simulink model "switch_5_24_TN0104"  (R2016b)
settings: Solver=VariableStepAuto  StartTime=0.0  StopTime=0.001  FixedStep=0.001  MaxStep=400e-9  RelTol=1e-3
libraries: fl_lib x9, nesl_utility x4, elec_lib x2
settings Model: Creator=piotr  LastModifiedBy=piotr

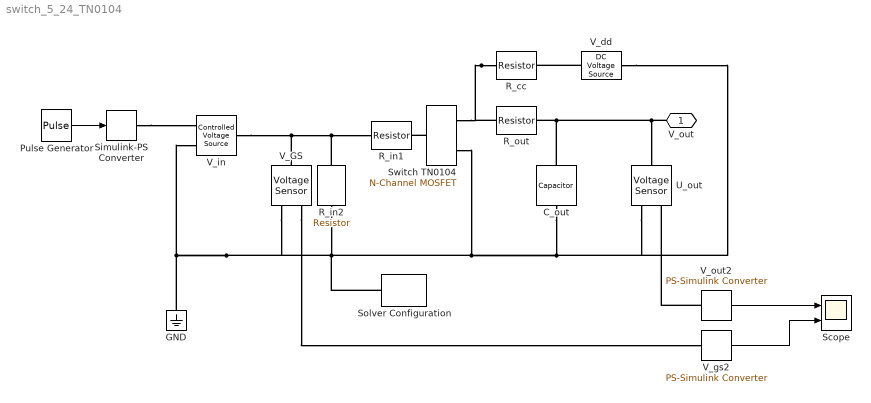
== system switch_5_24_TN0104 ==
  C_out : elec_lib/Passive Devices/Capacitor  enable_table=0  c=10 pF  Cvec=[ 1e-5 1e-6 ] F  Vvec=[ 0 10 ] V  CV_table_symmetry=1  C_tol=5  enable_C_tol=0  tol_distribution=1  nSigma=4  r=1e-6 Ohm  g=0 1/Ohm  initV=0 V  enable_operating_limits=0  operating_limit_action=2  max_working_voltage_range=[ -25 25 ] V  power_rating=1 W  enable_faults=0  fault_action=1  Cscale_faulted=100  R_faulted=0.001 Ohm  G_faulted=0 1/Ohm  tau_fault=0.001 s  enable_temporal_fault=0  t_fault=1 s  enable_behavioral_fault=0  max_permissible_voltage_range=[ -100 100 ] V  t_fail_on_voltage=1 s
  GND : fl_lib/Electrical/Electrical Elements/Electrical Reference
  Pulse Generator : DiscretePulseGenerator  PulseType=Time based  Amplitude=4.5  Period=0.0004  PulseWidth=50
  R_cc : fl_lib/Electrical/Electrical Elements/Resistor  R=2700 Ohm  i_specify=off  i_priority=None  i=0 A  v_specify=off  v_priority=None  v=0 V
  R_in1 : fl_lib/Electrical/Electrical Elements/Resistor  R=1 kOhm  i_specify=off  i_priority=None  i=0 A  v_specify=off  v_priority=None  v=0 V
  R_in2 : fl_lib/Electrical/Electrical Elements/Resistor  R=100 kOhm  i_specify=off  i_priority=None  i=0 A  v_specify=off  v_priority=None  v=0 V
  R_out : fl_lib/Electrical/Electrical Elements/Resistor  R=1 kOhm  i_specify=off  i_priority=None  i=0 A  v_specify=off  v_priority=None  v=0 V
  Scope : Scope  NumInputPorts=2
  Simulink-PS Converter : nesl_utility/Simulink-PS Converter  PhysicalDomain=network_engine_domain  SubClassName=ps_input  LeftPortType=input  RightPortType=output  PseudoPeriodic=off  Frequencies=[]  NoiseDistribution=none  NoiseParameters=[]  Unit=1  AffineConversion=off  InputFiltering=off  SimscapeFilterOrder=1  InputFilterTimeConstant=0.001  UdotUserProvided=1
  Solver Configuration : nesl_utility/Solver Configuration  PhysicalDomain=network_engine_domain  SubClassName=solver  LeftPortType=input  RightPortType=generic  Accelerate=off  Tones=[]  Harmonics=[]  SimulateNoise=off  Profile=off  UseLocalSampling=off  EnableSwitchedLinearOptims=on  FrequencyDomain=off  UseCCode=off  RelTol=0.001  AbsTol=1e-06  MinStep=1e-09  ToWorkspace=off  RevertToSquareIcSolve=off  NumHomotopyIterations=100  PhasorMode=off  PhasorModeNumHarmonics=1  OverrideAbsTol=off  DoDC=off  ResidualTolerance=1e-9  UseLocalSolver=off  LocalSolverChoice=NE_TRAPEZOIDAL_ADVANCER  LocalSolverSampleTime=0.0001  DoFixedCost=off  MaxNonlinIter=3  MaxModeIter=2  LinearAlgebra=Sparse  DelaysMemoryBudget=1024  AutomaticFiltering=on  FilteringTimeConstant=0.001
  Switch TN0104 : elec_lib/Semiconductor Devices/N-Channel MOSFET  parameterization=1  prmDatasheet=1  prmEquCoeff=1  Beta=5 A/V^2  Rds=1.5 Ohm  Id=1 A  Vgs=10 V  Vth=0.6 V  lam=0 1/V  Tmeas=25 degC  RS=1e-4 Ohm  RD=0.01 Ohm  C_param=1  C_GS=270 pF  C_GD=80 pF  C_DS=0 pF  C_iss=70 pF  C_rss=15 pF  C_oss=50 pF  C_GS_vec=[ 270 300 290 280 295 255 ] pF  C_GD_vec=[ 450 400 300 190 95 55 ] pF  C_DS_vec=[ 450 410 390 230 175 115 ] pF  C_iss_vec=[ 720 700 590 470 390 310 ] pF  C_rss_vec=[ 450 400 300 190 95 55 ] pF  C_oss_vec=[ 900 810 690 420 270 170 ] pF  C_Vds_vec=[ 0.1 0.3 1 3 10 30 ] V  charge_linearity_param=1  C_OX=200 pF  V_C_OX=-0.5 V  IsDiode=0 A  Vbi=0.6 V  n=1  Cj0Diode=10 pF  TT=50e-9 s  dVth_dT=-6 mV/K  Rds_T2=0.037 Ohm  Tmeas2=125 degC  BEXDatasheet=-1.5  BEXEquCoeff=-1.5  etaisDatasheet=3  etaisEquCoeff=3  TdeviceDatasheet=25 degC  TdeviceEquCoeff=25 degC  Rth=[1.0, 10.0] K/W  thermal_mass_parameterization=1  thermal_mass=[1.0, 1.0] J/K  thermal_time_constant=[1.0, 10.0] s  thermal_mass_initial_temperatures=[ 25 25 ] degC  betaref=18 A/V^2  Vfbref=-1.1 V  gamma=3.5 V^0.50000  phib2ref=1 V  thesatref=0.4 1/V  alpha=0  Vp=5e-2 V  m=8  Tref=25 degC  Cox=1500 pF  Cgso=100 pF  Cgdo=14 pF  Rsref=2e-3 Ohm  Rdref=0.17 Ohm  Rgref=8.4 Ohm  Isref=5.2e-13 A  Cj0=480 pF  Tprm=1  etabet=1.3  Stvfb=5e-4 V/K  Stphib=-8.5e-4 V/K  etasat=1.04  etar=0.95  etais=3  Tsim=25 degC  T0=[25.0, 25.0] degC
  U_out : fl_lib/Electrical/Electrical Sensors/Voltage Sensor
  V_GS : fl_lib/Electrical/Electrical Sensors/Voltage Sensor
  V_dd : fl_lib/Electrical/Electrical Sources/DC Voltage Source  v0=24 V
  V_gs2 : nesl_utility/PS-Simulink Converter  PhysicalDomain=network_engine_domain  SubClassName=ps_output  LeftPortType=input  RightPortType=output  PseudoPeriodic=off  Frequencies=[]  Unit=1  AffineConversion=off
  V_in : fl_lib/Electrical/Electrical Sources/Controlled Voltage Source
  V_out2 : nesl_utility/PS-Simulink Converter  PhysicalDomain=network_engine_domain  SubClassName=ps_output  LeftPortType=input  RightPortType=output  PseudoPeriodic=off  Frequencies=[]  Unit=1  AffineConversion=off
  V_out : PMIOPort  Port=1  Side=Left
  wires:
  Pulse Generator/1 -> Simulink-PS Converter/1
  V_out2/1 -> Scope/1
  V_gs2/1 -> Scope/2
  connections:
  Switch TN0104/LConn1 -- R_in1/RConn1
  Simulink-PS Converter/RConn1 -- V_in/RConn1
  V_dd/LConn1 -- R_cc/RConn1
  V_out2/LConn1 -- U_out/RConn1
  V_in/LConn1 -- V_GS/LConn1 -- R_in2/LConn1 -- R_in1/LConn1
  V_GS/RConn1 -- V_gs2/LConn1
  GND/LConn1 -- V_GS/RConn2 -- C_out/RConn1 -- V_dd/RConn1 -- U_out/RConn2 -- Switch TN0104/RConn2 -- Solver Configuration/RConn1 -- R_in2/RConn1 -- V_in/RConn2
  V_out/RConn1 -- R_out/RConn1 -- C_out/LConn1 -- U_out/LConn1
  R_cc/LConn1 -- Switch TN0104/RConn1 -- R_out/LConn1
